simulink model "AION_IDS_SPEEDGOAT"  (R2021a)
settings: configuration reference "AION_IDS_Speedgoat" (kept outside this file)
undefined symbols (not defined in the file): ADCU_SCU_CYCLE_TIME, AutoTrqWhlReq_test, BeamReq_test, BodyCtrlReq_test, BrakeReq_test, C, CONTROL_CYCLE_TIME, GearLvlReq_test, GearLvlReqVD_test, HornRingReq_test, LatCtrlReq_test, LngCtrlReq_test, SCU_ADCU_CYCLE_TIME, SteerAngReq_test, SteerWhlTorqReq_test, TurnLightReq_test
libraries: canmsglib x16, speedgoatlib_IO612 x5, simulink x1
settings Model: DataDictionary=AION_IDS.sldd  SimulationMode=external  ExtModeBatchMode=on  ExtModeTrigType=signal  Creator=xinrui  LastModifiedBy=Administrator
settings ConfigSetRef: SourceName=AION_IDS_Speedgoat

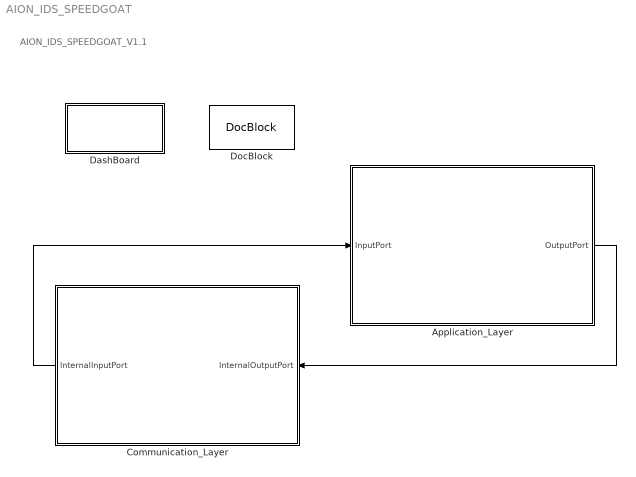
== system AION_IDS_SPEEDGOAT ==
  note: AION_IDS_SPEEDGOAT_V1.1
  Application_Layer : Subsystem
  Communication_Layer : Subsystem
  DashBoard : Subsystem
  DocBlock : simulink/Model-Wide Utilities/DocBlock  DocumentType=HTML  mask(DocBlock){}
      mask Display:
      | plot([.8 0 0 1 1 .8 .8 1],[1 1 0 0 .8 1 .8 .8]);
      | text(.5,.6,'CHANGELOG','horizontalalignment','center');
      | text(.95,.05,get_param(gcb,'DocumentType'),'verticalalignment','bottom','horizontalalignment','right');
  wires:
  Application_Layer/1(OutputPort) -> Communication_Layer/1(InternalOutputPort)
  Communication_Layer/1(InternalInputPort) -> Application_Layer/1(InputPort)

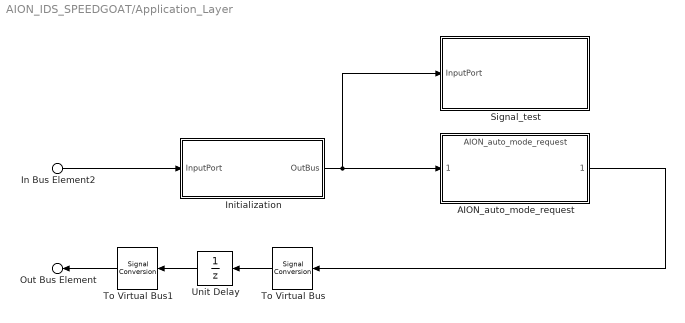
== system AION_IDS_SPEEDGOAT/Application_Layer ==
  In Bus Element2 : Inport  PortName=InputPort
  AION_auto_mode_request : ModelReference  ModelNameDialog=AION_auto_mode_request.slx  SimulationMode=Normal  ModelReferenceVersion=1.99
  Initialization : Subsystem
  Signal_test : Subsystem
  To Virtual Bus : SignalConversion  ConversionOutput=Nonvirtual bus  OutDataTypeStr=Bus: AION_ApplicationBus  OverrideOpt=off
  To Virtual Bus1 : SignalConversion  ConversionOutput=Virtual bus  OverrideOpt=off
  Unit Delay : UnitDelay  SampleTime=CONTROL_CYCLE_TIME  HasFrameUpgradeWarning=on
  Out Bus Element : Outport  PortName=OutputPort
  wires:
  To Virtual Bus/1 -> Unit Delay/1
  Unit Delay/1 -> To Virtual Bus1/1
  To Virtual Bus1/1 -> Out Bus Element/1
  AION_auto_mode_request/1 -> To Virtual Bus/1
  In Bus Element2/1 -> Initialization/1(InputPort)
  Initialization/1(OutBus) -> AION_auto_mode_request/1, Signal_test/1(InputPort)

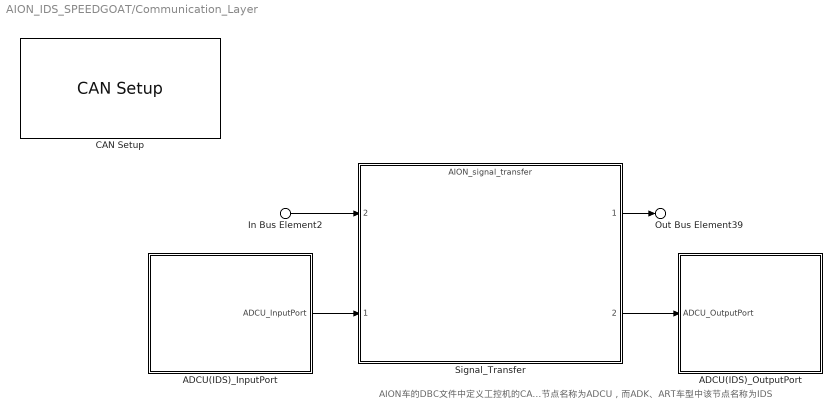
== system AION_IDS_SPEEDGOAT/Communication_Layer ==
  note: AION车的DBC文件中定义工控机的CAN节点名称为ADCU，而ADK、ART车型中该节点名称为IDS
  In Bus Element2 : Inport  PortName=InternalOutputPort
  ADCU(IDS)_InputPort : Subsystem
  ADCU(IDS)_OutputPort : Subsystem
  CAN Setup : speedgoatlib_IO612/CAN Setup  id=1  drvLtr=C:  PCISlot=-1  port1=CAN (HS)  port2=CAN (HS)  port3=Disable  port4=Disable  opModeCAN1=Highspeed (HS)  bdrCAN1=500 kBaud  usrBdrCAN1=[10, 1, 13, 2]  stdAccMaskCAN1=[0, 0]  extAccMaskCAN1=[0, 0]  opModeCAN2=Highspeed (HS)  bdrCAN2=500 kBaud  usrBdrCAN2=[10, 1, 13, 2]  stdAccMaskCAN2=[0, 0]  extAccMaskCAN2=[0, 0]  opModeCAN3=Highspeed (HS)  bdrCAN3=500 kBaud  usrBdrCAN3=[10, 1, 13, 2]  stdAccMaskCAN3=[0, 0]  extAccMaskCAN3=[0, 0]  opModeCAN4=Highspeed (HS)  bdrCAN4=500 kBaud  usrBdrCAN4=[10, 1, 13, 2]  stdAccMaskCAN4=[0, 0]  extAccMaskCAN4=[0, 0]  initStruct=[]  termStruct=[]  protl=IO612  qtyMod=1  chNo=[1, 2, 3, 4]  ptTypes=[1, 1, 1, 1]  protlHelpIdx=[0, 1, 2, 3]  isFDMod=0
      settings: SourceProductName=Simulink Real-Time: Speedgoat Library
  Signal_Transfer : ModelReference  ModelNameDialog=AION_signal_transfer.slx  SimulationMode=Normal  ModelReferenceVersion=4.87
      settings: PortSchema="{\"entries\":[{\"content\":{\"sides\":[{\"content\":{\"connectorIds\":[\"In2\",\"In1\"]},\"type\":\"ConnectorPlacement.EquallySpacedRectSide\",\"uuid\":\"d7b49387-9132-4f68-80a0-6c78bc11624f\"},{\"content\":{\"connectorIds\":[\"Out1\",\"Out2\"],\"side\":\"RIGHT\"},\"type\":\"ConnectorPlacement.EquallySpacedRectSide\",\"uuid\":\"3b80b3bd-44fe-4064-8909-e0d3ddc33b1d\"},{\"content\":{\"connectorIds\":[],\"side\":\"TOP\"},\"type\":\"ConnectorPlacement.EquallySpacedRectSide\",\"uuid\":\"9e6df871-f0e1-4d71-be51-8adc92933544\"}]},\"type\":\"ConnectorPlacement.EquallySpacedConnector\",\"uuid\":\"d7e504ac-b336-4965-bcb2-373027d2eba4\"}],\"packageUris\":[\"http://schema.mathworks.com/mf0/Connector/R2020b\"],\"version\":\"1.0\"}"
  Out Bus Element39 : Outport  PortName=InternalInputPort
  wires:
  Signal_Transfer/2 -> ADCU(IDS)_OutputPort/1(ADCU_OutputPort)
  In Bus Element2/1 -> Signal_Transfer/2
  ADCU(IDS)_InputPort/1(ADCU_InputPort) -> Signal_Transfer/1
  Signal_Transfer/1 -> Out Bus Element39/1

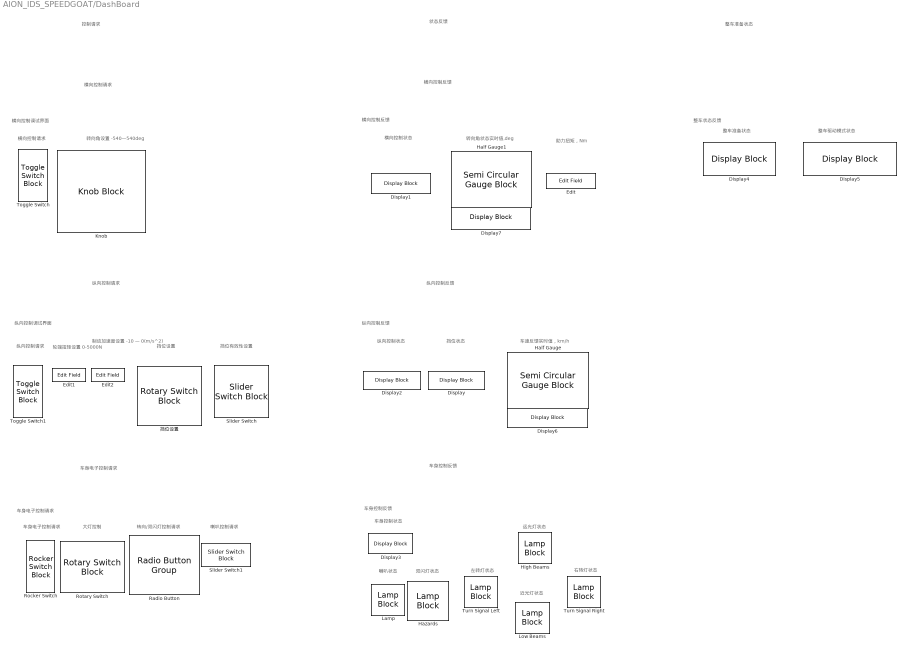
== system AION_IDS_SPEEDGOAT/DashBoard ==
  note: 纵向控制调试界面
  note: 横向控制调试界面
  note: 横向控制请求
  note: 纵向控制请求
  note: 挡位设置
  note: 挡位有效性设置
  note: 轮端扭矩设置
      | 0-5000N
  note: 制动加速度设置
      | -10 — 0(m/s^2)
  note: 转向角设置
      | -540—540deg
  note: 车身电子控制请求
  note: 整车状态反馈
  note: 车身电子控制请求
  note: 车身电子控制请求
  note: 纵向控制请求
  note: 横向控制请求
  note: 纵向控制反馈
  note: 大灯控制
  note: 转向/双闪灯控制请求
  note: 喇叭控制请求
  note: 控制请求
  note: 状态反馈
  note: 横向控制反馈
  note: 横向控制反馈
  note: 车身控制反馈
  note: 车身控制反馈
  note: 车速反馈实时值，km/h
  note: 纵向控制状态
  note: 挡位状态
  note: 横向控制状态
  note: 转向角状态实时值,deg
  note: 喇叭状态
  note: 左转灯状态
  note: 远光灯状态
  note: 右转灯状态
  note: 双闪灯状态
  note: 车身控制状态
  note: 近光灯状态
  note: 纵向控制反馈
  note: 整车准备状态
  note: 整车准备状态
  note: 整车驱动模式状态
  note: 助力扭矩，Nm
  Display{,1..7} (8 alike) : DisplayBlock  LabelPosition=Hide  Format=short  Transparency=1
  Edit : EditField  LabelPosition=Hide  ShowInitialText=on  Alignment=Center
  Edit1 : EditField  LabelPosition=Hide  ShowInitialText=on  Alignment=Center
  Edit2 : EditField  LabelPosition=Hide  ShowInitialText=on  Alignment=Center
  Half Gauge : SemiCircularGaugeBlock  ScaleMax=150
  Half Gauge1 : SemiCircularGaugeBlock  ScaleMin=-480  ScaleMax=480
  Hazards : LampBlock  Icon=Hazards
  High Beams : LampBlock  Icon=HighBeams
  Knob : KnobBlock  ScaleMin=-540  ScaleMax=540
  Lamp : LampBlock
  Low Beams : LampBlock  Icon=LowBeams
  Radio Button : RadioButtonGroup  SelectedLabel=No request  ButtonGroupName=Group
      settings: Values={{'No request', 'Turn left lig', 'Turn right light', 'Emergency light'}, [0 1 2 3]}
  Rocker Switch : RockerSwitchBlock
      settings: Values={{'Disable', 'Enable'}, [0 1]}
  Rotary Switch : RotarySwitchBlock
      settings: Values={{'OFF', 'Low', 'High'}, [0 1 2]}
  Slider Switch : SliderSwitchBlock
      settings: Values={{'Valid', 'Invalid'}, [1 0]}
  Slider Switch1 : SliderSwitchBlock
      settings: Values={{'Active', 'No active'}, [1 0]}
  Toggle Switch : ToggleSwitchBlock
      settings: Values={{'Manual', 'Auto'}, [0 1]}
  Toggle Switch1 : ToggleSwitchBlock
      settings: Values={{'Manual', 'Auto'}, [0 1]}
  Turn Signal Left : LampBlock  Icon=TurnSignalLeft
  Turn Signal Right : LampBlock  Icon=TurnSignalRight
  挡位设置 : RotarySwitchBlock
      settings: Values={{'No request', 'Park', 'Reversed', 'Neutral', 'Drive'}, [0 1 2 3 4]}

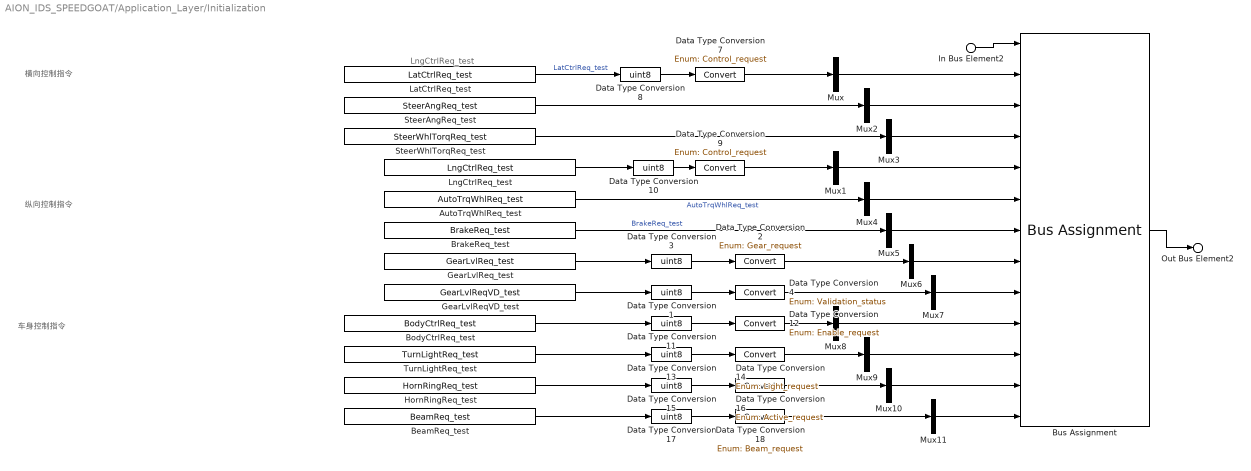
== system AION_IDS_SPEEDGOAT/Application_Layer/Initialization ==
  note: LngCtrlReq_test
  note: 横向控制指令
  note: 纵向控制指令
  note: 车身控制指令
  In Bus Element2 : Inport  PortName=InputPort
  AutoTrqWhlReq_test : Constant  Value=AutoTrqWhlReq_test  OutDataTypeStr=double  SampleTime=CONTROL_CYCLE_TIME
  BeamReq_test : Constant  Value=BeamReq_test  OutDataTypeStr=double  SampleTime=CONTROL_CYCLE_TIME
  BodyCtrlReq_test : Constant  Value=BodyCtrlReq_test  OutDataTypeStr=double  SampleTime=CONTROL_CYCLE_TIME
  BrakeReq_test : Constant  Value=BrakeReq_test  OutDataTypeStr=double  SampleTime=CONTROL_CYCLE_TIME
  Bus Assignment : BusAssignment  AssignedSignals=set_lateral_control_info.set_LatCtrlReq,set_lateral_control_info.set_SteerAngReq,set_lateral_control_info.set_SteerWhlTorqReq,set_longitudinal_control_info.set_LngCtrlReq,set_longitudinal_control_info.set_AutoTrqWhlReq,set_longitudinal_control_info.set_BrakeReq,set_longitudinal_control_info.set_GearLvlReq,set_longitudinal_control_info.set_GearLvlReqVD,set_ADCU_info.set_BodyCtrlReq,set_ADCU_info.set_TurnLightReq,set_ADCU_info.set_HornRingReq,set_ADCU_info.set_BeamReq
  Data Type Conversion{1,3,8,10..11,13,15,17} (8 alike) : DataTypeConversion  OutDataTypeStr=uint8
  Data Type Conversion12 : DataTypeConversion  OutDataTypeStr=Enum: Enable_request
  Data Type Conversion14 : DataTypeConversion  OutDataTypeStr=Enum: Light_request
  Data Type Conversion16 : DataTypeConversion  OutDataTypeStr=Enum: Active_request
  Data Type Conversion18 : DataTypeConversion  OutDataTypeStr=Enum: Beam_request
  Data Type Conversion2 : DataTypeConversion  OutDataTypeStr=Enum: Gear_request
  Data Type Conversion4 : DataTypeConversion  OutDataTypeStr=Enum: Validation_status
  Data Type Conversion7 : DataTypeConversion  OutDataTypeStr=Enum: Control_request
  Data Type Conversion9 : DataTypeConversion  OutDataTypeStr=Enum: Control_request
  GearLvlReqVD_test : Constant  Value=GearLvlReqVD_test  OutDataTypeStr=double  SampleTime=CONTROL_CYCLE_TIME
  GearLvlReq_test : Constant  Value=GearLvlReq_test  OutDataTypeStr=double  SampleTime=CONTROL_CYCLE_TIME
  HornRingReq_test : Constant  Value=HornRingReq_test  OutDataTypeStr=double  SampleTime=CONTROL_CYCLE_TIME
  LatCtrlReq_test : Constant  Value=LatCtrlReq_test  OutDataTypeStr=double  SampleTime=CONTROL_CYCLE_TIME
  LngCtrlReq_test : Constant  Value=LngCtrlReq_test  OutDataTypeStr=double  SampleTime=CONTROL_CYCLE_TIME
  Mux{,1..11} (12 alike) : Mux  Inputs=1
  SteerAngReq_test : Constant  Value=SteerAngReq_test  OutDataTypeStr=double  SampleTime=CONTROL_CYCLE_TIME
  SteerWhlTorqReq_test : Constant  Value=SteerWhlTorqReq_test  OutDataTypeStr=double  SampleTime=CONTROL_CYCLE_TIME
  TurnLightReq_test : Constant  Value=TurnLightReq_test  OutDataTypeStr=double  SampleTime=CONTROL_CYCLE_TIME
  Out Bus Element2 : Outport  PortName=OutBus
  wires:
  In Bus Element2/1 -> Bus Assignment/1
  Bus Assignment/1 -> Out Bus Element2/1
  Data Type Conversion9/1 -> Mux1/1
  Data Type Conversion10/1 -> Data Type Conversion9/1
  Data Type Conversion8/1 -> Data Type Conversion7/1
  LngCtrlReq_test/1 -> Data Type Conversion10/1
  GearLvlReq_test/1 -> Data Type Conversion3/1
  SteerAngReq_test/1 -> Mux2/1
  AutoTrqWhlReq_test/1 -> Mux4/1  "AutoTrqWhlReq_test"
  Data Type Conversion1/1 -> Data Type Conversion4/1
  GearLvlReqVD_test/1 -> Data Type Conversion1/1
  Data Type Conversion3/1 -> Data Type Conversion2/1
  BrakeReq_test/1 -> Mux5/1  "BrakeReq_test"
  Data Type Conversion2/1 -> Mux6/1
  Data Type Conversion4/1 -> Mux7/1
  LatCtrlReq_test/1 -> Data Type Conversion8/1  "LatCtrlReq_test"
  Mux7/1 -> Bus Assignment/9
  Mux6/1 -> Bus Assignment/8
  Mux2/1 -> Bus Assignment/3
  Mux1/1 -> Bus Assignment/5
  Mux/1 -> Bus Assignment/2
  Data Type Conversion12/1 -> Mux8/1
  Data Type Conversion11/1 -> Data Type Conversion12/1
  Data Type Conversion13/1 -> Data Type Conversion14/1
  Data Type Conversion14/1 -> Mux9/1
  Data Type Conversion16/1 -> Mux10/1
  Data Type Conversion15/1 -> Data Type Conversion16/1
  Data Type Conversion17/1 -> Data Type Conversion18/1
  Data Type Conversion18/1 -> Mux11/1
  BodyCtrlReq_test/1 -> Data Type Conversion11/1
  TurnLightReq_test/1 -> Data Type Conversion13/1
  HornRingReq_test/1 -> Data Type Conversion15/1
  BeamReq_test/1 -> Data Type Conversion17/1
  Mux11/1 -> Bus Assignment/13
  Mux10/1 -> Bus Assignment/12
  Mux9/1 -> Bus Assignment/11
  Mux8/1 -> Bus Assignment/10
  Mux4/1 -> Bus Assignment/6
  Mux5/1 -> Bus Assignment/7
  Data Type Conversion7/1 -> Mux/1
  Mux3/1 -> Bus Assignment/4
  SteerWhlTorqReq_test/1 -> Mux3/1

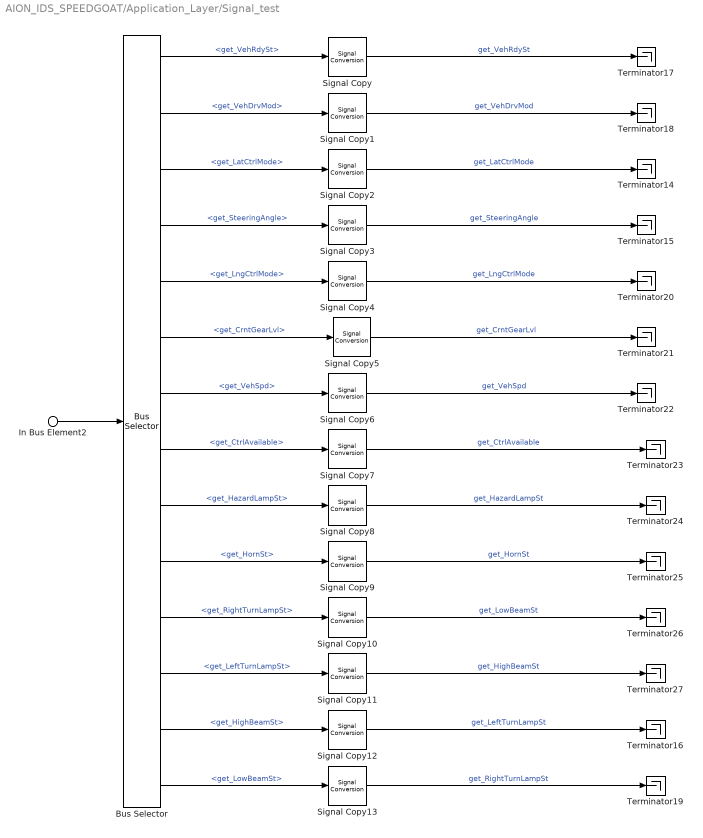
== system AION_IDS_SPEEDGOAT/Application_Layer/Signal_test ==
  In Bus Element2 : Inport  PortName=InputPort
  Bus Selector : BusSelector  OutputSignals=get_VCU_info.get_VehRdySt,get_VCU_info.get_VehDrvMod,get_SCU_info.get_LatCtrlMode,get_EPS_info.get_SteeringAngle,get_SCU_info.get_LngCtrlMode,get_VCU_info.get_CrntGearLvl,get_BCS_info.get_VehSpd,get_BCM_info.get_CtrlAvailable,get_BCM_info.get_HazardLampSt,get_BCM_info.get_HornSt,get_BCM_info.get_RightTurnLampSt,get_BCM_info.get_LeftTurnLampSt,get_BCM_info.get_HighBeamSt,get_BCM_info.get_LowBeamSt
  Signal Copy{,1..13} (14 alike) : SignalConversion  OverrideOpt=off
  Terminator{14..27} (14 alike) : Terminator
  wires:
  Signal Copy7/1 -> Terminator23/1  "get_CtrlAvailable"
  Signal Copy2/1 -> Terminator14/1  "get_LatCtrlMode"
  Signal Copy6/1 -> Terminator22/1  "get_VehSpd"
  Signal Copy/1 -> Terminator17/1  "get_VehRdySt"
  Signal Copy5/1 -> Terminator21/1  "get_CrntGearLvl"
  Signal Copy8/1 -> Terminator24/1  "get_HazardLampSt"
  Signal Copy9/1 -> Terminator25/1  "get_HornSt"
  Signal Copy3/1 -> Terminator15/1  "get_SteeringAngle"
  Signal Copy10/1 -> Terminator26/1  "get_LowBeamSt"
  Signal Copy4/1 -> Terminator20/1  "get_LngCtrlMode"
  Signal Copy1/1 -> Terminator18/1  "get_VehDrvMod"
  Signal Copy11/1 -> Terminator27/1  "get_HighBeamSt"
  Signal Copy12/1 -> Terminator16/1  "get_LeftTurnLampSt"
  Signal Copy13/1 -> Terminator19/1  "get_RightTurnLampSt"
  In Bus Element2/1 -> Bus Selector/1
  Bus Selector/8 -> Signal Copy7/1  "<get_CtrlAvailable>"
  Bus Selector/9 -> Signal Copy8/1  "<get_HazardLampSt>"
  Bus Selector/10 -> Signal Copy9/1  "<get_HornSt>"
  Bus Selector/3 -> Signal Copy2/1  "<get_LatCtrlMode>"
  Bus Selector/4 -> Signal Copy3/1  "<get_SteeringAngle>"
  Bus Selector/5 -> Signal Copy4/1  "<get_LngCtrlMode>"
  Bus Selector/12 -> Signal Copy11/1  "<get_LeftTurnLampSt>"
  Bus Selector/13 -> Signal Copy12/1  "<get_HighBeamSt>"
  Bus Selector/14 -> Signal Copy13/1  "<get_LowBeamSt>"
  Bus Selector/7 -> Signal Copy6/1  "<get_VehSpd>"
  Bus Selector/2 -> Signal Copy1/1  "<get_VehDrvMod>"
  Bus Selector/6 -> Signal Copy5/1  "<get_CrntGearLvl>"
  Bus Selector/11 -> Signal Copy10/1  "<get_RightTurnLampSt>"
  Bus Selector/1 -> Signal Copy/1  "<get_VehRdySt>"

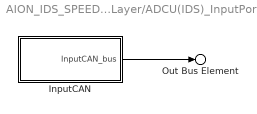
== system AION_IDS_SPEEDGOAT/Communication_Layer/ADCU(IDS)_InputPort ==
  InputCAN : Subsystem
  Out Bus Element : Outport  PortName=ADCU_InputPort  Element=InputCAN_bus
  wires:
  InputCAN/1(InputCAN_bus) -> Out Bus Element/1

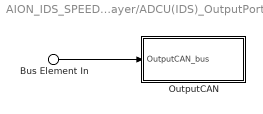
== system AION_IDS_SPEEDGOAT/Communication_Layer/ADCU(IDS)_OutputPort ==
  Bus Element In : Inport  PortName=ADCU_OutputPort  Element=OutputCAN_bus
  OutputCAN : Subsystem
  wires:
  Bus Element In/1 -> OutputCAN/1(OutputCAN_bus)

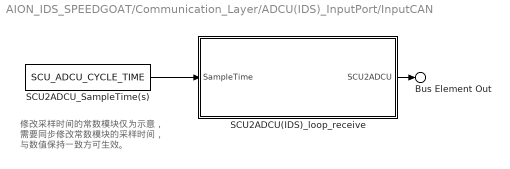
== system AION_IDS_SPEEDGOAT/Communication_Layer/ADCU(IDS)_InputPort/InputCAN ==
  note: 修改采样时间的常数模块仅为示意，
      | 需要同步修改常数模块的采样时间，
      | 与数值保持一致方可生效。
  SCU2ADCU(IDS)_loop_receive : Subsystem  TreatAsAtomicUnit=on
  SCU2ADCU_SampleTime(s) : Constant  Value=SCU_ADCU_CYCLE_TIME  SampleTime=ADCU_SCU_CYCLE_TIME
  Bus Element Out : Outport  PortName=InputCAN_bus  Element=SCU2ADCU_bus
  wires:
  SCU2ADCU_SampleTime(s)/1 -> SCU2ADCU(IDS)_loop_receive/1(SampleTime)
  SCU2ADCU(IDS)_loop_receive/1(SCU2ADCU) -> Bus Element Out/1

== system AION_IDS_SPEEDGOAT/Communication_Layer/ADCU(IDS)_OutputPort/OutputCAN ==
  Bus Element In : Inport  PortName=OutputCAN_bus  Element=ADCU2SCU_bus
  CAN_pack_ADCU2SCU : Subsystem
  wires:
  Bus Element In/1 -> CAN_pack_ADCU2SCU/1(ADCU2SCU)

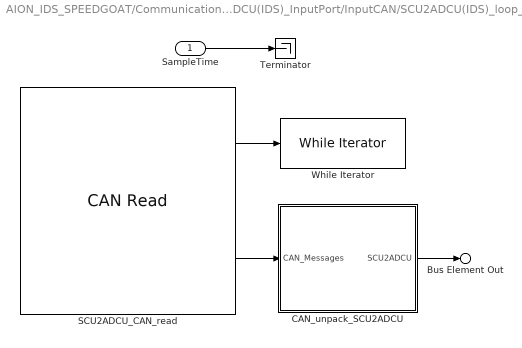
== system AION_IDS_SPEEDGOAT/Communication_Layer/ADCU(IDS)_InputPort/InputCAN/SCU2ADCU(IDS)_loop_receive ==
  SampleTime : Inport
  CAN_unpack_SCU2ADCU : Subsystem
  SCU2ADCU_CAN_read : speedgoatlib_IO612/CAN Read  id=1  sampleTime=-1  portSelection=1  messageType=CAN  protl=IO612  ptIdx=0  isFDMod=0
      settings: SourceProductName=Simulink Real-Time: Speedgoat Library
  Terminator : Terminator
  While Iterator : WhileIterator  MaxIters=-1  WhileBlockType=do-while
  Bus Element Out : Outport  PortName=SCU2ADCU
  wires:
  SCU2ADCU_CAN_read/1 -> While Iterator/1
  CAN_unpack_SCU2ADCU/1(SCU2ADCU) -> Bus Element Out/1
  SCU2ADCU_CAN_read/2 -> CAN_unpack_SCU2ADCU/1(CAN_Messages)
  SampleTime/1 -> Terminator/1

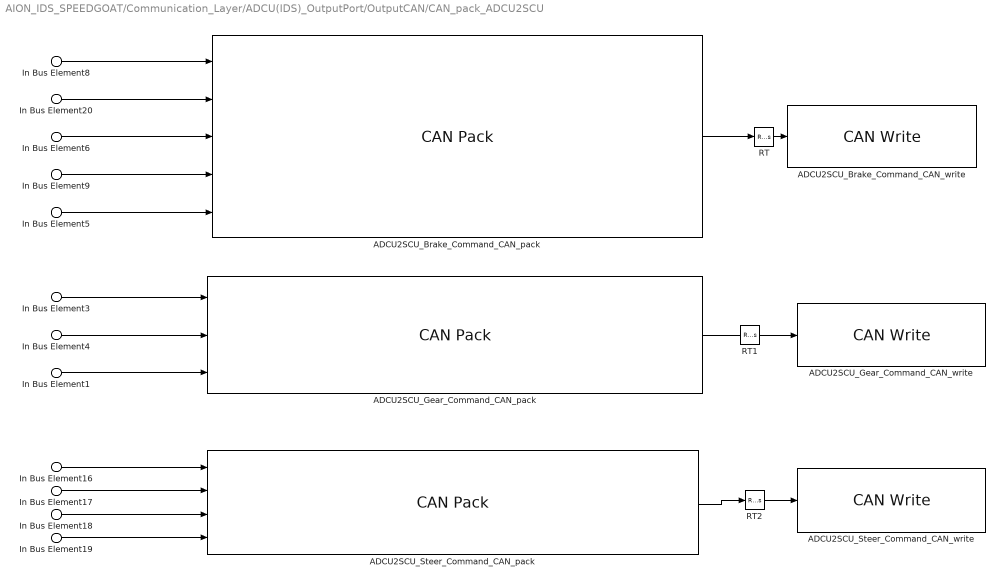
== system AION_IDS_SPEEDGOAT/Communication_Layer/ADCU(IDS)_OutputPort/OutputCAN/CAN_pack_ADCU2SCU ==
  In Bus Element8 : Inport  PortName=ADCU2SCU  Element=ADCU_1.ADCU_AutoTrqWhlReq
  In Bus Element20 : Inport  PortName=ADCU2SCU  Element=ADCU_1.ADCU_BrakeReq
  In Bus Element6 : Inport  PortName=ADCU2SCU  Element=ADCU_1.ADCU_GearLvlReq
  In Bus Element9 : Inport  PortName=ADCU2SCU  Element=ADCU_1.ADCU_GearLvlReqVD
  In Bus Element5 : Inport  PortName=ADCU2SCU  Element=ADCU_1.ADCU_LngCtrlReq
  In Bus Element3 : Inport  PortName=ADCU2SCU  Element=ADCU_2.ADCU_LatCtrlReq
  In Bus Element4 : Inport  PortName=ADCU2SCU  Element=ADCU_2.ADCU_SteerAngReq
  In Bus Element1 : Inport  PortName=ADCU2SCU  Element=ADCU_2.ADCU_SteerWhlTorqReq
  In Bus Element16 : Inport  PortName=ADCU2SCU  Element=ADCU_3.ADCU_BeamReq
  In Bus Element17 : Inport  PortName=ADCU2SCU  Element=ADCU_3.ADCU_BodyCtrlReq
  In Bus Element18 : Inport  PortName=ADCU2SCU  Element=ADCU_3.ADCU_HornRingReq
  In Bus Element19 : Inport  PortName=ADCU2SCU  Element=ADCU_3.ADCU_TurnLightReq
  ADCU2SCU_Brake_Command_CAN_pack : canmsglib/CAN Pack  CANdbFile=data\DBC\AION_ADCU.dbc  MsgList=ADCU_1  MsgName=ADCU_1  MsgIDType=Standard (11-bit identifier)  MsgIdentifier=544  MsgLength=8  Remote=off  ApplyMinMax=off  BusOutput=off  SignalInfo={'ADCU_AutoTrqWhlReq','26','14','BE','unsigned','Standard','0','1','-5000','-5000','5000';'ADCU_BrakeReq','8','16','BE','unsigned','Standard','0','0.0004882','-16','-16','16';'ADCU_GearLvlReq','37','3','BE','unsigned','Standard','0','1','0','0','7';'ADCU_GearLvlReqVD','36','1','BE','unsigned','Standard','0','1','0','0','1';'ADCU_LngCtrlReq','24','2','BE','unsigned','Standard','0','1','0','0','3'}
      settings: SourceProductBaseCode=ME,XP,VN  DataFormat=CANdb specified signals
  ADCU2SCU_Brake_Command_CAN_write : speedgoatlib_IO612/CAN Write  id=1  sampleTime=ADCU_SCU_CYCLE_TIME  portSelection=1  messageType=CAN  enaStatusPort=off  protl=IO612  ptIdx=0  isFDMod=0
      settings: SourceProductName=Simulink Real-Time: Speedgoat Library
  ADCU2SCU_Gear_Command_CAN_pack : canmsglib/CAN Pack  CANdbFile=data\DBC\AION_ADCU.dbc  MsgList=ADCU_2  MsgName=ADCU_2  MsgIDType=Standard (11-bit identifier)  MsgIdentifier=545  MsgLength=8  Remote=off  ApplyMinMax=off  BusOutput=off  SignalInfo={'ADCU_LatCtrlReq','44','1','BE','unsigned','Standard','0','1','0','0','1';'ADCU_SteerAngReq','8','16','BE','unsigned','Standard','0','0.1','-780','-780','779.9';'ADCU_SteerWhlTorqReq','45','11','BE','unsigned','Standard','0','0.01','-10.24','-10.24','10.23'}
      settings: SourceProductBaseCode=ME,XP,VN  DataFormat=CANdb specified signals
  ADCU2SCU_Gear_Command_CAN_write : speedgoatlib_IO612/CAN Write  id=1  sampleTime=ADCU_SCU_CYCLE_TIME  portSelection=1  messageType=CAN  enaStatusPort=off  protl=IO612  ptIdx=0  isFDMod=0
      settings: SourceProductName=Simulink Real-Time: Speedgoat Library
  ADCU2SCU_Steer_Command_CAN_pack : canmsglib/CAN Pack  CANdbFile=data\DBC\AION_ADCU.dbc  MsgList=ADCU_3  MsgName=ADCU_3  MsgIDType=Standard (11-bit identifier)  MsgIdentifier=640  MsgLength=8  Remote=off  ApplyMinMax=off  BusOutput=off  SignalInfo={'ADCU_BeamReq','2','2','BE','unsigned','Standard','0','1','0','0','3';'ADCU_BodyCtrlReq','4','1','BE','unsigned','Standard','0','1','0','0','1';'ADCU_HornRingReq','5','1','BE','unsigned','Standard','0','1','0','0','1';'ADCU_TurnLightReq','0','2','BE','unsigned','Standard','0','1','0','0','3'}
      settings: SourceProductBaseCode=ME,XP,VN  DataFormat=CANdb specified signals
  ADCU2SCU_Steer_Command_CAN_write : speedgoatlib_IO612/CAN Write  id=1  sampleTime=ADCU3_SCU_CYCLE_TIME  portSelection=1  messageType=CAN  enaStatusPort=off  protl=IO612  ptIdx=0  isFDMod=0
      settings: SourceProductName=Simulink Real-Time: Speedgoat Library
  RT : RateTransition  Deterministic=off  OutPortSampleTime=0.02
  RT1 : RateTransition  Deterministic=off  OutPortSampleTime=0.02
  RT2 : RateTransition  Deterministic=off  OutPortSampleTime=0.05
  wires:
  RT/1 -> ADCU2SCU_Brake_Command_CAN_write/1
  RT1/1 -> ADCU2SCU_Gear_Command_CAN_write/1
  RT2/1 -> ADCU2SCU_Steer_Command_CAN_write/1
  ADCU2SCU_Gear_Command_CAN_pack/1 -> RT1/1
  ADCU2SCU_Brake_Command_CAN_pack/1 -> RT/1
  ADCU2SCU_Steer_Command_CAN_pack/1 -> RT2/1
  In Bus Element8/1 -> ADCU2SCU_Brake_Command_CAN_pack/1
  In Bus Element20/1 -> ADCU2SCU_Brake_Command_CAN_pack/2
  In Bus Element6/1 -> ADCU2SCU_Brake_Command_CAN_pack/3
  In Bus Element9/1 -> ADCU2SCU_Brake_Command_CAN_pack/4
  In Bus Element5/1 -> ADCU2SCU_Brake_Command_CAN_pack/5
  In Bus Element3/1 -> ADCU2SCU_Gear_Command_CAN_pack/1
  In Bus Element4/1 -> ADCU2SCU_Gear_Command_CAN_pack/2
  In Bus Element16/1 -> ADCU2SCU_Steer_Command_CAN_pack/1
  In Bus Element17/1 -> ADCU2SCU_Steer_Command_CAN_pack/2
  In Bus Element18/1 -> ADCU2SCU_Steer_Command_CAN_pack/3
  In Bus Element19/1 -> ADCU2SCU_Steer_Command_CAN_pack/4
  In Bus Element1/1 -> ADCU2SCU_Gear_Command_CAN_pack/3

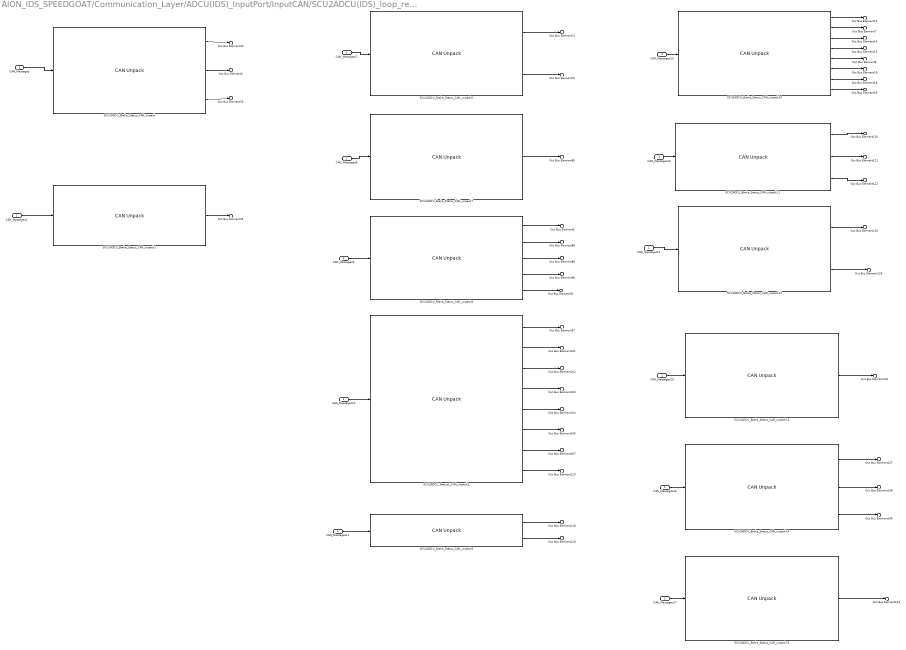
== system AION_IDS_SPEEDGOAT/Communication_Layer/ADCU(IDS)_InputPort/InputCAN/SCU2ADCU(IDS)_loop_receive/CAN_unpack_SCU2ADCU ==
  CAN_Messages : Inport
  CAN_Messages{2,7..17} (12 alike) : InportShadow
  SCU2ADCU_Brake_Status_CAN_unpack : canmsglib/CAN Unpack  CANdbFile=data\DBC\AION_ADCU.dbc  MsgList=SCU_1  MsgName=SCU_1  MsgIDType=Standard (11-bit identifier)  MsgIdentifier=384  MsgLength=8  SignalInfo={'BCS_ABSActiveSt','1','1','BE','unsigned','Standard','0','1','0','0','1';'BCS_VehSpd','40','13','BE','unsigned','Standard','0','0.05625','0','0','240';'BCS_VehSpdVD','37','1','BE','unsigned','Standard','0','1','0','0','1'}  IDPort=off  TimestampPort=off  ErrorPort=off  RemotePort=off  LengthPort=off  StatusPort=off  ApplyMinMax=off
      settings: SourceProductBaseCode=ME,XP,VN  DataFormat=CANdb specified signals
  SCU2ADCU_Brake_Status_CAN_unpack1 : canmsglib/CAN Unpack  CANdbFile=data\DBC\AION_ADCU.dbc  MsgList=SCU_3  MsgName=SCU_3  MsgIDType=Standard (11-bit identifier)  MsgIdentifier=547  MsgLength=8  SignalInfo={'BCS_YawRate','8','12','BE','unsigned','Standard','0','0.00097656','-2.0943','-2.0943','1.9047'}  IDPort=off  TimestampPort=off  ErrorPort=off  RemotePort=off  LengthPort=off  StatusPort=off  ApplyMinMax=off
      settings: SourceProductBaseCode=ME,XP,VN  DataFormat=CANdb specified signals
  SCU2ADCU_Brake_Status_CAN_unpack10 : canmsglib/CAN Unpack  CANdbFile=data\DBC\AION_ADCU.dbc  MsgList=SCU_13  MsgName=SCU_13  MsgIDType=Standard (11-bit identifier)  MsgIdentifier=554  MsgLength=8  SignalInfo={'SCU_LatAutoCheckReport','52','4','BE','unsigned','Standard','0','1','0','0','15';'SCU_LatCtrlMode','2','2','BE','unsigned','Standard','0','1','0','0','3';'SCU_LatQuitReport','24','8','BE','unsigned','Standard','0','1','0','0','255';'SCU_LngAutoChecklReport','40','16','BE','unsigned','Standard','0','1','0','0','65535';'SCU_LngCtrlMode','0','2','BE','unsigned','Standard','0','1','0','0','3';'SCU_LngQuitReport','16','16','BE','unsigned','Standard','0','1','0','0','65535';'SCU_StrngWhlIntv','7','1','BE','unsigned','Standard','0','1','0','0','1';'VCU_GearLeverIntv','6','1','BE','unsigned','Standard','0','1','0','0','1'}  IDPort=off  TimestampPort=off  ErrorPort=off  RemotePort=off  LengthPort=off  StatusPort=off  ApplyMinMax=off
      settings: SourceProductBaseCode=ME,XP,VN  DataFormat=CANdb specified signals
  SCU2ADCU_Brake_Status_CAN_unpack11 : canmsglib/CAN Unpack  CANdbFile=data\DBC\AION_ADCU.dbc  MsgList=SCU_14  MsgName=SCU_14  MsgIDType=Standard (11-bit identifier)  MsgIdentifier=706  MsgLength=8  SignalInfo={'VCU_VehDrvMod','11','3','BE','unsigned','Standard','0','1','0','0','7';'VCU_VehRdySt','10','1','BE','unsigned','Standard','0','1','0','0','1';'VCU_VehRng','14','10','BE','unsigned','Standard','0','1','0','0','1000'}  IDPort=off  TimestampPort=off  ErrorPort=off  RemotePort=off  LengthPort=off  StatusPort=off  ApplyMinMax=off
      settings: SourceProductBaseCode=ME,XP,VN  DataFormat=CANdb specified signals
  SCU2ADCU_Brake_Status_CAN_unpack12 : canmsglib/CAN Unpack  CANdbFile=data\DBC\AION_ADCU.dbc  MsgList=SCU_15  MsgName=SCU_15  MsgIDType=Standard (11-bit identifier)  MsgIdentifier=555  MsgLength=8  SignalInfo={'VCU_CrntGearLvl','36','3','BE','unsigned','Standard','0','1','0','0','7';'VCU_CrntGearLvlVD','35','1','BE','unsigned','Standard','0','1','0','0','1'}  IDPort=off  TimestampPort=off  ErrorPort=off  RemotePort=off  LengthPort=off  StatusPort=off  ApplyMinMax=off
      settings: SourceProductBaseCode=ME,XP,VN  DataFormat=CANdb specified signals
  SCU2ADCU_Brake_Status_CAN_unpack13 : canmsglib/CAN Unpack  CANdbFile=data\DBC\AION_ADCU.dbc  MsgList=SCU_16  MsgName=SCU_16  MsgIDType=Standard (11-bit identifier)  MsgIdentifier=556  MsgLength=8  SignalInfo={'VCU_ActVehWheelTorq','42','14','BE','unsigned','Standard','0','1','0','0','10000'}  IDPort=off  TimestampPort=off  ErrorPort=off  RemotePort=off  LengthPort=off  StatusPort=off  ApplyMinMax=off
      settings: SourceProductBaseCode=ME,XP,VN  DataFormat=CANdb specified signals
  SCU2ADCU_Brake_Status_CAN_unpack14 : canmsglib/CAN Unpack  CANdbFile=data\DBC\AION_ADCU.dbc  MsgList=SCU_17  MsgName=SCU_17  MsgIDType=Standard (11-bit identifier)  MsgIdentifier=557  MsgLength=8  SignalInfo={'VCU_AccElecECFail','30','1','BE','unsigned','Standard','0','1','0','0','1';'VCU_GasPedalActPst','40','8','BE','unsigned','Standard','0','0.392','0','0','99.96';'VCU_VehWheelTorqMax','10','14','BE','unsigned','Standard','0','1','0','0','10000'}  IDPort=off  TimestampPort=off  ErrorPort=off  RemotePort=off  LengthPort=off  StatusPort=off  ApplyMinMax=off
      settings: SourceProductBaseCode=ME,XP,VN  DataFormat=CANdb specified signals
  SCU2ADCU_Brake_Status_CAN_unpack15 : canmsglib/CAN Unpack  CANdbFile=data\DBC\AION_ADCU.dbc  MsgList=SCU_18  MsgName=SCU_18  MsgIDType=Standard (11-bit identifier)  MsgIdentifier=559  MsgLength=8  SignalInfo={'VCU_BrkPedalSt','53','1','BE','unsigned','Standard','0','1','0','0','1'}  IDPort=off  TimestampPort=off  ErrorPort=off  RemotePort=off  LengthPort=off  StatusPort=off  ApplyMinMax=off
      settings: SourceProductBaseCode=ME,XP,VN  DataFormat=CANdb specified signals
  SCU2ADCU_Brake_Status_CAN_unpack6 : canmsglib/CAN Unpack  CANdbFile=data\DBC\AION_ADCU.dbc  MsgList=SCU_8  MsgName=SCU_8  MsgIDType=Standard (11-bit identifier)  MsgIdentifier=551  MsgLength=8  SignalInfo={'BCS_ActVehLaltrlAccel','36','12','BE','unsigned','Standard','0','0.027127','-21.593','-21.593','21.593';'BCS_ActVehLongAccel','12','12','BE','unsigned','Standard','0','0.027127','-21.593','-21.593','21.593'}  IDPort=off  TimestampPort=off  ErrorPort=off  RemotePort=off  LengthPort=off  StatusPort=off  ApplyMinMax=off
      settings: SourceProductBaseCode=ME,XP,VN  DataFormat=CANdb specified signals
  SCU2ADCU_Brake_Status_CAN_unpack7 : canmsglib/CAN Unpack  CANdbFile=data\DBC\AION_ADCU.dbc  MsgList=SCU_9  MsgName=SCU_9  MsgIDType=Standard (11-bit identifier)  MsgIdentifier=552  MsgLength=8  SignalInfo={'EPB_SysSt','8','3','BE','unsigned','Standard','0','1','0','0','7'}  IDPort=off  TimestampPort=off  ErrorPort=off  RemotePort=off  LengthPort=off  StatusPort=off  ApplyMinMax=off
      settings: SourceProductBaseCode=ME,XP,VN  DataFormat=CANdb specified signals
  SCU2ADCU_Brake_Status_CAN_unpack8 : canmsglib/CAN Unpack  CANdbFile=data\DBC\AION_ADCU.dbc  MsgList=SCU_10  MsgName=SCU_10  MsgIDType=Standard (11-bit identifier)  MsgIdentifier=553  MsgLength=8  SignalInfo={'EPS_SteeringAngle','16','16','BE','unsigned','Standard','0','0.1','-780','-780','779.9';'EPS_SteeringAngleSpd','38','8','BE','unsigned','Standard','0','4','0','0','1016';'EPS_SteeringAngleSpdVD','7','1','BE','unsigned','Standard','0','1','0','0','1';'EPS_SteeringAngleVD','34','1','BE','unsigned','Standard','0','1','0','0','1';'EPS_StrngWhlTorq','40','8','BE','unsigned','Standard','0','0.1','-12.7','-12.5','12.5'}  IDPort=off  TimestampPort=off  ErrorPort=off  RemotePort=off  LengthPort=off  StatusPort=off  ApplyMinMax=off
      settings: SourceProductBaseCode=ME,XP,VN  DataFormat=CANdb specified signals
  SCU2ADCU_Brake_Status_CAN_unpack9 : canmsglib/CAN Unpack  CANdbFile=data\DBC\AION_ADCU.dbc  MsgList=SCU_12  MsgName=SCU_12  MsgIDType=Standard (11-bit identifier)  MsgIdentifier=705  MsgLength=8  SignalInfo={'SRS_DriverSeatBeltSt','2','2','BE','unsigned','Standard','0','1','0','0','3';'SRS_PsngrSeatBeltSt','0','2','BE','unsigned','Standard','0','1','0','0','3'}  IDPort=off  TimestampPort=off  ErrorPort=off  RemotePort=off  LengthPort=off  StatusPort=off  ApplyMinMax=off
      settings: SourceProductBaseCode=ME,XP,VN  DataFormat=CANdb specified signals
  SCU2ADCU_Status1_CAN_unpack1 : canmsglib/CAN Unpack  CANdbFile=data\DBC\AION_ADCU.dbc  MsgList=SCU_11  MsgName=SCU_11  MsgIDType=Standard (11-bit identifier)  MsgIdentifier=704  MsgLength=8  SignalInfo={'BCM_CtrlAvailable','18','1','BE','unsigned','Standard','0','1','0','0','1';'BCM_HazardLampSt','16','1','BE','unsigned','Standard','0','1','0','0','1';'BCM_HighBeamSt','5','1','BE','unsigned','Standard','0','1','0','0','1';'BCM_HornSt','17','1','BE','unsigned','Standard','0','1','0','0','1';'BCM_KeySt','2','2','BE','unsigned','Standard','0','1','0','0','3';'BCM_LeftTurnLampSt','12','1','BE','unsigned','Standard','0','1','0','0','1';'BCM_LowBeamSt','4','1','BE','unsigned','Standard','0','1','0','0','1';'BCM_RightTurnLampSt','14','1','BE','unsigned','Standard','0','1','0','0','1'}  IDPort=off  TimestampPort=off  ErrorPort=off  RemotePort=off  LengthPort=off  StatusPort=off  ApplyMinMax=off
      settings: SourceProductBaseCode=ME,XP,VN  DataFormat=CANdb specified signals
  Out Bus Element20 : Outport  PortName=SCU2ADCU  Element=SCU_1.BCS_ABSActiveSt
  Out Bus Element5 : Outport  PortName=SCU2ADCU  Element=SCU_1.BCS_VehSpd
  Out Bus Element23 : Outport  PortName=SCU2ADCU  Element=SCU_1.BCS_VehSpdVD
  Out Bus Element6 : Outport  PortName=SCU2ADCU  Element=SCU_10.EPS_SteeringAngle
  Out Bus Element88 : Outport  PortName=SCU2ADCU  Element=SCU_10.EPS_SteeringAngleSpd
  Out Bus Element89 : Outport  PortName=SCU2ADCU  Element=SCU_10.EPS_SteeringAngleSpdVD
  Out Bus Element90 : Outport  PortName=SCU2ADCU  Element=SCU_10.EPS_SteeringAngleVD
  Out Bus Element91 : Outport  PortName=SCU2ADCU  Element=SCU_10.EPS_StrngWhlTorq
  Out Bus Element97 : Outport  PortName=SCU2ADCU  Element=SCU_11.BCM_CtrlAvailable
  Out Bus Element101 : Outport  PortName=SCU2ADCU  Element=SCU_11.BCM_HazardLampSt
  Out Bus Element102 : Outport  PortName=SCU2ADCU  Element=SCU_11.BCM_HighBeamSt
  Out Bus Element103 : Outport  PortName=SCU2ADCU  Element=SCU_11.BCM_HornSt
  Out Bus Element104 : Outport  PortName=SCU2ADCU  Element=SCU_11.BCM_KeySt
  Out Bus Element106 : Outport  PortName=SCU2ADCU  Element=SCU_11.BCM_LeftTurnLampSt
  Out Bus Element107 : Outport  PortName=SCU2ADCU  Element=SCU_11.BCM_LowBeamSt
  Out Bus Element113 : Outport  PortName=SCU2ADCU  Element=SCU_11.BCM_RightTurnLampSt
  Out Bus Element118 : Outport  PortName=SCU2ADCU  Element=SCU_12.SRS_DriverSeatBeltSt
  Out Bus Element119 : Outport  PortName=SCU2ADCU  Element=SCU_12.SRS_PsngrSeatBeltSt
  Out Bus Element13 : Outport  PortName=SCU2ADCU  Element=SCU_13.SCU_LatAutoCheckReport
  Out Bus Element7 : Outport  PortName=SCU2ADCU  Element=SCU_13.SCU_LatCtrlMode
  Out Bus Element14 : Outport  PortName=SCU2ADCU  Element=SCU_13.SCU_LatQuitReport
  Out Bus Element15 : Outport  PortName=SCU2ADCU  Element=SCU_13.SCU_LngAutoChecklReport
  Out Bus Element8 : Outport  PortName=SCU2ADCU  Element=SCU_13.SCU_LngCtrlMode
  Out Bus Element16 : Outport  PortName=SCU2ADCU  Element=SCU_13.SCU_LngQuitReport
  Out Bus Element18 : Outport  PortName=SCU2ADCU  Element=SCU_13.SCU_StrngWhlIntv
  Out Bus Element19 : Outport  PortName=SCU2ADCU  Element=SCU_13.VCU_GearLeverIntv
  Out Bus Element120 : Outport  PortName=SCU2ADCU  Element=SCU_14.VCU_VehDrvMod
  Out Bus Element121 : Outport  PortName=SCU2ADCU  Element=SCU_14.VCU_VehRdySt
  Out Bus Element122 : Outport  PortName=SCU2ADCU  Element=SCU_14.VCU_VehRng
  Out Bus Element125 : Outport  PortName=SCU2ADCU  Element=SCU_15.VCU_CrntGearLvl
  Out Bus Element126 : Outport  PortName=SCU2ADCU  Element=SCU_15.VCU_CrntGearLvlVD
  Out Bus Element131 : Outport  PortName=SCU2ADCU  Element=SCU_16.VCU_ActVehWheelTorq
  Out Bus Element137 : Outport  PortName=SCU2ADCU  Element=SCU_17.VCU_AccElecECFail
  Out Bus Element138 : Outport  PortName=SCU2ADCU  Element=SCU_17.VCU_GasPedalActPst
  Out Bus Element140 : Outport  PortName=SCU2ADCU  Element=SCU_17.VCU_VehWheelTorqMax
  Out Bus Element143 : Outport  PortName=SCU2ADCU  Element=SCU_18.VCU_BrkPedalSt
  Out Bus Element35 : Outport  PortName=SCU2ADCU  Element=SCU_3.BCS_YawRate
  Out Bus Element74 : Outport  PortName=SCU2ADCU  Element=SCU_8.BCS_ActVehLaltrlAccel
  Out Bus Element76 : Outport  PortName=SCU2ADCU  Element=SCU_8.BCS_ActVehLongAccel
  Out Bus Element85 : Outport  PortName=SCU2ADCU  Element=SCU_9.EPB_SysSt
  wires:
  CAN_Messages/1 -> SCU2ADCU_Brake_Status_CAN_unpack/1
  CAN_Messages2/1 -> SCU2ADCU_Brake_Status_CAN_unpack1/1
  SCU2ADCU_Brake_Status_CAN_unpack1/1 -> Out Bus Element35/1
  CAN_Messages7/1 -> SCU2ADCU_Brake_Status_CAN_unpack6/1
  CAN_Messages8/1 -> SCU2ADCU_Brake_Status_CAN_unpack7/1
  CAN_Messages12/1 -> SCU2ADCU_Brake_Status_CAN_unpack10/1
  CAN_Messages17/1 -> SCU2ADCU_Brake_Status_CAN_unpack15/1
  CAN_Messages13/1 -> SCU2ADCU_Brake_Status_CAN_unpack11/1
  CAN_Messages14/1 -> SCU2ADCU_Brake_Status_CAN_unpack12/1
  CAN_Messages11/1 -> SCU2ADCU_Brake_Status_CAN_unpack9/1
  CAN_Messages15/1 -> SCU2ADCU_Brake_Status_CAN_unpack13/1
  CAN_Messages9/1 -> SCU2ADCU_Brake_Status_CAN_unpack8/1
  CAN_Messages16/1 -> SCU2ADCU_Brake_Status_CAN_unpack14/1
  CAN_Messages10/1 -> SCU2ADCU_Status1_CAN_unpack1/1
  SCU2ADCU_Brake_Status_CAN_unpack6/1 -> Out Bus Element74/1
  SCU2ADCU_Brake_Status_CAN_unpack11/2 -> Out Bus Element121/1
  SCU2ADCU_Brake_Status_CAN_unpack11/1 -> Out Bus Element120/1
  SCU2ADCU_Brake_Status_CAN_unpack11/3 -> Out Bus Element122/1
  SCU2ADCU_Brake_Status_CAN_unpack/1 -> Out Bus Element20/1
  SCU2ADCU_Brake_Status_CAN_unpack/2 -> Out Bus Element5/1
  SCU2ADCU_Brake_Status_CAN_unpack/3 -> Out Bus Element23/1
  SCU2ADCU_Brake_Status_CAN_unpack6/2 -> Out Bus Element76/1
  SCU2ADCU_Brake_Status_CAN_unpack7/1 -> Out Bus Element85/1
  SCU2ADCU_Brake_Status_CAN_unpack8/5 -> Out Bus Element91/1
  SCU2ADCU_Brake_Status_CAN_unpack8/1 -> Out Bus Element6/1
  SCU2ADCU_Brake_Status_CAN_unpack8/2 -> Out Bus Element88/1
  SCU2ADCU_Brake_Status_CAN_unpack8/3 -> Out Bus Element89/1
  SCU2ADCU_Brake_Status_CAN_unpack8/4 -> Out Bus Element90/1
  SCU2ADCU_Status1_CAN_unpack1/1 -> Out Bus Element97/1
  SCU2ADCU_Status1_CAN_unpack1/2 -> Out Bus Element101/1
  SCU2ADCU_Status1_CAN_unpack1/3 -> Out Bus Element102/1
  SCU2ADCU_Status1_CAN_unpack1/4 -> Out Bus Element103/1
  SCU2ADCU_Status1_CAN_unpack1/5 -> Out Bus Element104/1
  SCU2ADCU_Status1_CAN_unpack1/6 -> Out Bus Element106/1
  SCU2ADCU_Status1_CAN_unpack1/7 -> Out Bus Element107/1
  SCU2ADCU_Status1_CAN_unpack1/8 -> Out Bus Element113/1
  SCU2ADCU_Brake_Status_CAN_unpack9/1 -> Out Bus Element118/1
  SCU2ADCU_Brake_Status_CAN_unpack9/2 -> Out Bus Element119/1
  SCU2ADCU_Brake_Status_CAN_unpack10/1 -> Out Bus Element13/1
  SCU2ADCU_Brake_Status_CAN_unpack10/2 -> Out Bus Element7/1
  SCU2ADCU_Brake_Status_CAN_unpack10/3 -> Out Bus Element14/1
  SCU2ADCU_Brake_Status_CAN_unpack10/4 -> Out Bus Element15/1
  SCU2ADCU_Brake_Status_CAN_unpack10/5 -> Out Bus Element8/1
  SCU2ADCU_Brake_Status_CAN_unpack10/6 -> Out Bus Element16/1
  SCU2ADCU_Brake_Status_CAN_unpack10/7 -> Out Bus Element18/1
  SCU2ADCU_Brake_Status_CAN_unpack10/8 -> Out Bus Element19/1
  SCU2ADCU_Brake_Status_CAN_unpack12/1 -> Out Bus Element125/1
  SCU2ADCU_Brake_Status_CAN_unpack12/2 -> Out Bus Element126/1
  SCU2ADCU_Brake_Status_CAN_unpack13/1 -> Out Bus Element131/1
  SCU2ADCU_Brake_Status_CAN_unpack14/1 -> Out Bus Element137/1
  SCU2ADCU_Brake_Status_CAN_unpack14/2 -> Out Bus Element138/1
  SCU2ADCU_Brake_Status_CAN_unpack14/3 -> Out Bus Element140/1
  SCU2ADCU_Brake_Status_CAN_unpack15/1 -> Out Bus Element143/1
